simulink model "Intergration"  (R2018b)
settings: Solver=FixedStepDiscrete  StartTime=0.0  StopTime=inf  FixedStep=0.005  RelTol=1e-3
PostLoadFcn:
  | if any(exist('dsrtsu_mdlpostloadfcn', 'file') ~= 0), dsrtsu_mdlpostloadfcn('Execute', bdroot); end
values from neighbouring files (symbols this model uses):
  P_x165_On = 1.0    [CAN_Tx.sldd]
  P_x242_On = 1.0    [CAN_Tx.sldd]
  P_x246_On = 1.0    [CAN_Tx.sldd]
libraries: rtican x112, simulink x59
(part 4 of 31)

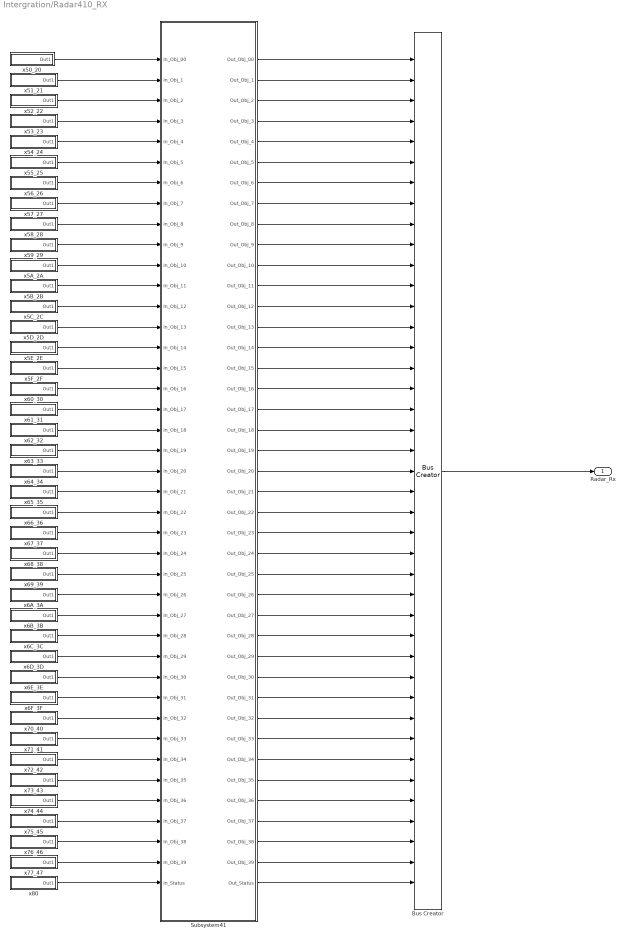
== system Intergration/Radar410_RX ==
  Bus Creator : BusCreator  Inputs=41  OutDataTypeStr=Bus: Radar410_Info_ST  NonVirtualBus=on
      settings: InheritFromInputs=off
  Subsystem41 : Subsystem
  x50_20 : Subsystem
  x51_21 : Subsystem
  x52_22 : Subsystem
  x53_23 : Subsystem
  x54_24 : Subsystem
  x55_25 : Subsystem
  x56_26 : Subsystem
  x57_27 : Subsystem
  x58_28 : Subsystem
  x59_29 : Subsystem
  x5A_2A : Subsystem
  x5B_2B : Subsystem
  x5C_2C : Subsystem
  x5D_2D : Subsystem
  x5E_2E : Subsystem
  x5F_2F : Subsystem
  x60_30 : Subsystem
  x61_31 : Subsystem
  x62_32 : Subsystem
  x63_33 : Subsystem
  x64_34 : Subsystem
  x65_35 : Subsystem
  x66_36 : Subsystem
  x67_37 : Subsystem
  x68_38 : Subsystem
  x69_39 : Subsystem
  x6A_3A : Subsystem
  x6B_3B : Subsystem
  x6C_3C : Subsystem
  x6D_3D : Subsystem
  x6E_3E : Subsystem
  x6F_3F : Subsystem
  x70_40 : Subsystem
  x71_41 : Subsystem
  x72_42 : Subsystem
  x73_43 : Subsystem
  x74_44 : Subsystem
  x75_45 : Subsystem
  x76_46 : Subsystem
  x77_47 : Subsystem
  x80 : Subsystem
  Radar_Rx : Outport  OutDataTypeStr=Bus: Radar410_Info_ST
  wires:
  Subsystem41/3(Out_Obj_2) -> Bus Creator/3
  x53_23/1(Out1) -> Subsystem41/4(In_Obj_3)
  x73_43/1(Out1) -> Subsystem41/36(In_Obj_35)
  x61_31/1(Out1) -> Subsystem41/18(In_Obj_17)
  x71_41/1(Out1) -> Subsystem41/34(In_Obj_33)
  x68_38/1(Out1) -> Subsystem41/25(In_Obj_24)
  Subsystem41/6(Out_Obj_5) -> Bus Creator/6
  Subsystem41/15(Out_Obj_14) -> Bus Creator/15
  Subsystem41/16(Out_Obj_15) -> Bus Creator/16
  Subsystem41/20(Out_Obj_19) -> Bus Creator/20
  x52_22/1(Out1) -> Subsystem41/3(In_Obj_2)
  Subsystem41/28(Out_Obj_27) -> Bus Creator/28
  Bus Creator/1 -> Radar_Rx/1
  Subsystem41/12(Out_Obj_11) -> Bus Creator/12
  x58_28/1(Out1) -> Subsystem41/9(In_Obj_8)
  Subsystem41/13(Out_Obj_12) -> Bus Creator/13
  Subsystem41/2(Out_Obj_1) -> Bus Creator/2
  x76_46/1(Out1) -> Subsystem41/39(In_Obj_38)
  Subsystem41/5(Out_Obj_4) -> Bus Creator/5
  x57_27/1(Out1) -> Subsystem41/8(In_Obj_7)
  x55_25/1(Out1) -> Subsystem41/6(In_Obj_5)
  x54_24/1(Out1) -> Subsystem41/5(In_Obj_4)
  x60_30/1(Out1) -> Subsystem41/17(In_Obj_16)
  x5A_2A/1(Out1) -> Subsystem41/11(In_Obj_10)
  Subsystem41/32(Out_Obj_31) -> Bus Creator/32
  x67_37/1(Out1) -> Subsystem41/24(In_Obj_23)
  x69_39/1(Out1) -> Subsystem41/26(In_Obj_25)
  x6C_3C/1(Out1) -> Subsystem41/29(In_Obj_28)
  x56_26/1(Out1) -> Subsystem41/7(In_Obj_6)
  x66_36/1(Out1) -> Subsystem41/23(In_Obj_22)
  x5F_2F/1(Out1) -> Subsystem41/16(In_Obj_15)
  x80/1(Out1) -> Subsystem41/41(In_Status)
  Subsystem41/41(Out_Status) -> Bus Creator/41
  x5E_2E/1(Out1) -> Subsystem41/15(In_Obj_14)
  x64_34/1(Out1) -> Subsystem41/21(In_Obj_20)
  x6F_3F/1(Out1) -> Subsystem41/32(In_Obj_31)
  x63_33/1(Out1) -> Subsystem41/20(In_Obj_19)
  Subsystem41/14(Out_Obj_13) -> Bus Creator/14
  x51_21/1(Out1) -> Subsystem41/2(In_Obj_1)
  Subsystem41/39(Out_Obj_38) -> Bus Creator/39
  x62_32/1(Out1) -> Subsystem41/19(In_Obj_18)
  x5B_2B/1(Out1) -> Subsystem41/12(In_Obj_11)
  Subsystem41/8(Out_Obj_7) -> Bus Creator/8
  Subsystem41/18(Out_Obj_17) -> Bus Creator/18
  Subsystem41/10(Out_Obj_9) -> Bus Creator/10
  x5C_2C/1(Out1) -> Subsystem41/13(In_Obj_12)
  Subsystem41/21(Out_Obj_20) -> Bus Creator/21
  x70_40/1(Out1) -> Subsystem41/33(In_Obj_32)
  x75_45/1(Out1) -> Subsystem41/38(In_Obj_37)
  x72_42/1(Out1) -> Subsystem41/35(In_Obj_34)
  Subsystem41/27(Out_Obj_26) -> Bus Creator/27
  Subsystem41/1(Out_Obj_00) -> Bus Creator/1
  x65_35/1(Out1) -> Subsystem41/22(In_Obj_21)
  Subsystem41/7(Out_Obj_6) -> Bus Creator/7
  Subsystem41/19(Out_Obj_18) -> Bus Creator/19
  Subsystem41/11(Out_Obj_10) -> Bus Creator/11
  x50_20/1(Out1) -> Subsystem41/1(In_Obj_00)
  x77_47/1(Out1) -> Subsystem41/40(In_Obj_39)
  x6B_3B/1(Out1) -> Subsystem41/28(In_Obj_27)
  Subsystem41/33(Out_Obj_32) -> Bus Creator/33
  Subsystem41/31(Out_Obj_30) -> Bus Creator/31
  Subsystem41/40(Out_Obj_39) -> Bus Creator/40
  x6A_3A/1(Out1) -> Subsystem41/27(In_Obj_26)
  Subsystem41/26(Out_Obj_25) -> Bus Creator/26
  Subsystem41/24(Out_Obj_23) -> Bus Creator/24
  x6D_3D/1(Out1) -> Subsystem41/30(In_Obj_29)
  Subsystem41/36(Out_Obj_35) -> Bus Creator/36
  Subsystem41/22(Out_Obj_21) -> Bus Creator/22
  Subsystem41/34(Out_Obj_33) -> Bus Creator/34
  Subsystem41/23(Out_Obj_22) -> Bus Creator/23
  Subsystem41/29(Out_Obj_28) -> Bus Creator/29
  Subsystem41/25(Out_Obj_24) -> Bus Creator/25
  Subsystem41/17(Out_Obj_16) -> Bus Creator/17
  Subsystem41/37(Out_Obj_36) -> Bus Creator/37
  x74_44/1(Out1) -> Subsystem41/37(In_Obj_36)
  x59_29/1(Out1) -> Subsystem41/10(In_Obj_9)
  x5D_2D/1(Out1) -> Subsystem41/14(In_Obj_13)
  Subsystem41/30(Out_Obj_29) -> Bus Creator/30
  Subsystem41/9(Out_Obj_8) -> Bus Creator/9
  Subsystem41/38(Out_Obj_37) -> Bus Creator/38
  Subsystem41/4(Out_Obj_3) -> Bus Creator/4
  x6E_3E/1(Out1) -> Subsystem41/31(In_Obj_30)
  Subsystem41/35(Out_Obj_34) -> Bus Creator/35

== system Intergration/TX ==
  VLC_LgtCmd_st : Inport  OutDataTypeStr=Bus: VLC_LGTCMD_ST  BusOutputAsStruct=on
  ACC_LgtCtrl_st : Inport  Port=2  OutDataTypeStr=Bus: ACC_LGTCTRL_ST  BusOutputAsStruct=on
  ATS_Po_st : Inport  Port=3  OutDataTypeStr=Bus: ATS_PO_ST
  COM_VehBus_st : Inport  Port=4
  do_20ms : TriggerPort  TriggerType=function-call  VariantControl=Variant
  Adapter_Tx : Subsystem
  Bus Selector : BusSelector  OutputSignals=x251.VehSdslSts,x24C.WhlGndVelLDrvn_Radar,x24C.WhlGndVelRDrvn_Radar,x24C.LDrvnWhlRotlDircn,x24C.RDrvnWhlRotlDircn,x24E.WhlGndVelLNonDrvn_Radar,x24E.WhlGndVelRNonDrvn_Radar,x24E.LNonDrvnWhlRotlDircn_Radar,x24E.RNonDrvnWhlRotlDircn_Radar,x23C.VehSpdAvg,x185.VSELongtAcc,x1E9.VehDynYawRate,x185.VSELatAcc
  Constant : Constant  Value=9.8
  Constant1 : Constant  Value=9.8
  Divide : Product  Inputs=*/
  Divide1 : Product  Inputs=*/
  ESC_DA_MESSAGE_0x127 : Subsystem
  ESC_FrontWheelSpeedKPH_0x123 : Subsystem
  ESC_RearWheelSpeedKPH_0x124 : Subsystem
  ESC_Status_0x126 : Subsystem
  RADAR_HSC2_FVCM_FrP00_0x165 : Subsystem
  RADAR_HSC2_FrP00_0x242 : Subsystem
  RADAR_HSC2_FrP01_0x244 : Subsystem
  RADAR_HSC2_FrP02_0x246 : Subsystem
  RollingCounter : Subsystem
  YRS1_0x131 : Subsystem
  YRS2_0x132 : Subsystem
  wires:
  VLC_LgtCmd_st/1 -> Adapter_Tx/1(VLC_LgtCmd_st)  "VLC_LgtCmd_st"
  RollingCounter/1(RC) -> RADAR_HSC2_FVCM_FrP00_0x165/1(RC), RADAR_HSC2_FrP01_0x244/1(RC), RADAR_HSC2_FrP00_0x242/1(RC)
  ATS_Po_st/1 -> Adapter_Tx/3(ATS_Po_st)
  ACC_LgtCtrl_st/1 -> Adapter_Tx/2(ACC_LgtCtrl_st)
  Adapter_Tx/3(x246) -> RADAR_HSC2_FrP02_0x246/1(COM_x246_st)
  Adapter_Tx/2(x165) -> RADAR_HSC2_FVCM_FrP00_0x165/2(COM_x165_st)  "COM_x165_st"
  Adapter_Tx/1(x242) -> RADAR_HSC2_FrP00_0x242/2(COM_x242_st)  "COM_x242_st"
  Bus Selector/8 -> ESC_RearWheelSpeedKPH_0x124/3(<LNonDrvnWhlRotlDircn_Radar>)  "<LNonDrvnWhlRotlDircn_Radar>"
  Constant/1 -> Divide/2
  Bus Selector/3 -> ESC_FrontWheelSpeedKPH_0x123/2(<WhlGndVelRDrvn_Radar>)  "<WhlGndVelRDrvn_Radar>"
  Constant1/1 -> Divide1/2
  Bus Selector/12 -> YRS1_0x131/1(<VehDynYawRate>)  "<VehDynYawRate>"
  COM_VehBus_st/1 -> Bus Selector/1
  Bus Selector/11 -> Divide/1  "<VSELongtAcc>"
  Divide1/1 -> YRS1_0x131/2(In2)
  Bus Selector/10 -> ESC_Status_0x126/1(<VehSpdAvg>)  "<VehSpdAvg>"
  Divide/1 -> YRS2_0x132/1(In1)
  Bus Selector/9 -> ESC_RearWheelSpeedKPH_0x124/4(<RNonDrvnWhlRotlDircn_Radar>)  "<RNonDrvnWhlRotlDircn_Radar>"
  Bus Selector/4 -> ESC_FrontWheelSpeedKPH_0x123/3(<LDrvnWhlRotlDircn>)  "<LDrvnWhlRotlDircn>"
  Bus Selector/13 -> Divide1/1  "<VSELatAcc>"
  Bus Selector/6 -> ESC_RearWheelSpeedKPH_0x124/1(<WhlGndVelLNonDrvn_Radar>)  "<WhlGndVelLNonDrvn_Radar>"
  Bus Selector/5 -> ESC_FrontWheelSpeedKPH_0x123/4(<RDrvnWhlRotlDircn>)  "<RDrvnWhlRotlDircn>"
  Bus Selector/7 -> ESC_RearWheelSpeedKPH_0x124/2(<WhlGndVelRNonDrvn_Radar>)  "<WhlGndVelRNonDrvn_Radar>"
  Bus Selector/2 -> ESC_FrontWheelSpeedKPH_0x123/1(<WhlGndVelLDrvn_Radar>)  "<WhlGndVelLDrvn_Radar>"
  Bus Selector/1 -> ESC_DA_MESSAGE_0x127/1(VehSdslStsHSC2)  "<VehSdslSts>"

== system Intergration/Tx_410_10ms ==
  COM_VehBus_st : Inport  OutDataTypeStr=Bus: COM_VEHBUS_ST  BusOutputAsStruct=on
  do_10ms : TriggerPort  TriggerType=function-call  VariantControl=Variant
  Abs : Abs
  Bus Selector1 : BusSelector  OutputSignals=x1E5.StrgWhlAngGrd,x1E5.StrgWhlAng
  Cast To Double{1..4} (4 alike) : DataTypeConversion  OutDataTypeStr=double
  Constant : Constant  Value=0  OutDataTypeStr=uint8
  Constant1 : Constant  Value=0  OutDataTypeStr=double
  Constant6 : Constant  Value=7  OutDataTypeStr=uint8
  RollingCounter1 : Subsystem
  S-Function Builder1 : S-Function  InitFcn=try, set_param(gcb,'FunctionName','CheckSum_Tx_Radar410'), end  FunctionName=CheckSum_Tx_Radar410  SFunctionModules=CheckSum_Tx_Radar410_wrapper  SFunctionDeploymentMode=off  EnableBusSupport=off  mask(S-Function Builder){}
      mask help: Simulink:masks:SFunctionBuilder_MD
      mask init:
      | val = [[.9  0.75 0.75 1 1 .9 .9 1]',[1 1 0.75 0.75 .9 .9 1 .9]'];try , sys = get_param(gcb,'SfunBuilderFcnName');if isempty(sys), sys = get_param(gcb,'FunctionName'); end,catch, sys = get_param(gcb,'FunctionName'); end
      settings: CopyFcn=set_param(gcbh,'LinkStatus','none')  PreSaveFcn=try, set_param(gcb,'FunctionName','CheckSum_Tx_Radar410'), end  OpenFcn=sfunctionwizard(gcbh)
      mask Display: plot(val(:,1),val(:,2)),disp(sys), port_label('input',1,'data'), port_label('input',2,'length'), port_label('output',1,'u8_crc8')
  SAS_Status : rtican/RTICAN Transmit (TX)   Reserved1=[]  Reserved2=[]  Reserved3=[]  Reserved4=[]  SfcnMessage=[]  Msg_Struct=[]  BoardTypeNo=[]  BoardNo=[]  ChannelNo=[]  Parameters=[]  DialogFcn=[]  UnitName=[]  Revision=[]  UnitValues=[]  DSProperties=struct('RTI',struct('Version',uint32(5),'BlockType',struct('isSLSource',uint8(1),'isSLSink',uint8(1),'isHWSource',uint8(0),'isHWSink',uint8(0),'isSetup',uint8(0),'isInline',uint8(1),'isNonInline',uint8(0),'isInterrupt',uint8(0),'isChannelwise',uint8(0)),'IOBoardType','RTICAN','UnitType','MESSAGE','Identifier','TX','DialogType','MSVC','BlockSet','RTICAN','SlaveProcessor','CAN'))  RTIBlockInterface=struct('InputPortsWidth',int32([1 1 1 1 1 1]),'InputPortsActive',[1 1 1 1 1 1],'InputPortsName',{{'SAS_Status_Checksum','SAS_Status_AliveCounter','SAS_CalibrationSts','SAS_FailureSts','SAS_SteerWheelRotSpd','SAS_SteerWheelAngle'}},'InputPortsDataType',{{'SS_DOUBLE','SS_DOUBLE','SS_DOUBLE','SS_DOUBLE','SS_DOUBLE','SS_DOUBLE'}},'OutputPortsWidth',int32([1 1 1 1]),'OutputPortsActive',[1 1 1 1],'OutputPortsName',{{['TX status'],['TX time'],['TX delta time'],['TX delay time']}},'DialogFcn','rtican_message_interface_gui','BlockDisplay',{{'','center'}},'IconTransparency','on','InitLevel',3,'BlockName',struct('Token',{{'SAS_Status'}}),'SampleTime',{{-1}},'TriggerPort',{{'none'}},'EnablePort',{{'none'}})  RTIBlockParameters=struct('BoardTypeNo',{{1,'OFF',[]}},'BoardNo',{{3,'ON',[1 16]}},'ChannelNo',{{2,'ON',[1 2]}},'Parameters',{{struct('DataFileSupport',struct('DataFileSelectedMaster',1,'DataFileSelectedLocal',1,'DataFileName','c:\users\administrator.zx-201607042142\documents\matlab\zone\dbc\ars410od_privatecan.dbc|c:\users\administrator.zx-201607042142\desktop\zone\2020_demo\410\asr410od_public_can.dbc|','DataFileDate',{{{''},{['30-十一月-2020 09:38:41']}}},'SelectedFile','..\..\..\..\..\desktop\zone\2020_demo\410\asr410od_public_can.dbc','InterfaceFcn','rtican_dbc_file_parser'),'Options',struct('StatusSelected',1,'TimeSelected',1,'DeltaTimeSelected',1,'DelayTimeSelected',1,'DelayTimeTXCommandSelected',0,'EncodeSetUnusedBitsToOne',0,'EnableMsgLoopback',0,'TriggerPort',struct('Selected',0,'TriggerType',0),'EnablePortSelected',0,'SignalOnPortnameSelected',1,'UserCoding',struct('Selected',0,'InterfaceFile','UserEncodingFile','FcnName','UserEncodeFcn','InportSelected',0,'InportWidth',1,'OutportSelected',0,'OutportWidth',1),'TerminationMsg',struct('Selected',0,'Byte0_7','0'),'InitialMsg',struct('Selected',0,'Byte0_7','0')),'Message',struct('MsgOnBlocknameSelected',1,'MsgName','SAS_Status','MsgIdFormat',0,'MsgId',225,'MsgLength',8,'NumSignals',6,'SampleTime',-1,'StartTime',struct('Selected',0,'Value',3),'AutoRepeatTime',struct('Selected',0,'Value',0.1),'Timeout',struct('Selected',0,'Value',0.1),'DelayTime',struct('Selected',0,'Value',0.1),'Signal',struct('SgnName',{'SAS_Status_Checksum','SAS_Status_AliveCounter','SAS_CalibrationSts','SAS_FailureSts','SAS_SteerWheelRotSpd','SAS_SteerWheelAngle'},'SgnStartBit',{16,28,38,39,40,48},'SgnLength',{8,4,1,1,8,16},'SgnType',{0,0,0,0,0,0},'ModeValue',{-1,-1,-1,-1,-1,-1},'DataType',{0,0,0,0,0,0},'ByteLayout',{2,2,2,2,2,2},'Factor',{1,1,1,1,4,0.1},'Offset',{0,0,0,0,0,-780},'SgnComment',{{'SAS_Status_Checksum'},{'SAS_Status_AliveCounter'},{'SAS_CalibrationSts'},{'SAS_FailureSts'},{'SAS_SteerWheelRotSpd'},{'SAS_SteerWheelAngle'}},'SgnUnit',{'','','','','',''},'Min',{0,0,0,0,0,-780},'Max',{255,15,1,1,1016,779.9},'SLDataType',{'SS_DOUBLE','SS_DOUBLE','SS_DOUBLE','SS_DOUBLE','SS_DOUBLE','SS_DOUBLE'}),'MsgIdNumFormat',1,'MsgComment',{{''}}),'Version',1.2,'general',struct('isFromLib',0)),'OFF',[]}},'GroupId',{{struct('Group',{{'RTICAN'}},'No',3,'Behavior',{{'NAMECHANGE'}},'BlockType',{{'SINK'}},'NameChangeFlag',0),'OFF',[]}},'SFcnRTICANMessage',{{struct('MsgType','TX','SFcnPortType','Scalar','MsgName','SAS_Status','MsgIdFormat','STD','MsgId',225,'MsgLength',8,'NumSignals',6,'SampleTime',-1,'StartTime',struct('Selected','no','Value',3),'AutoRepeatTime',struct('Selected','no','Value',0.1),'Timeout',struct('Selected','no','Value',0.1),'Signal',struct('SgnName',{'SAS_Status_Checksum','SAS_Status_AliveCounter','SAS_CalibrationSts','SAS_FailureSts','SAS_SteerWheelRotSpd','SAS_SteerWheelAngle'},'SgnStartBit',{16,28,38,39,40,48},'SgnLength',{8,4,1,1,8,16},'SgnType',{'standard','standard','standard','standard','standard','standard'},'ModeValue',{-1,-1,-1,-1,-1,-1},'DataType',{['unsigned int'],['unsigned int'],['unsigned int'],['unsigned int'],['unsigned int'],['unsigned int']},'ByteLayout',{['motorola back.'],['motorola back.'],['motorola back.'],['motorola back.'],['motorola back.'],['motorola back.']},'Factor',{1,1,1,1,4,0.1},'Offset',{0,0,0,0,0,-780},'SLDataType',{'SS_DOUBLE','SS_DOUBLE','SS_DOUBLE','SS_DOUBLE','SS_DOUBLE','SS_DOUBLE'}),'StatusSelected','yes','TimeSelected','yes','DeltaTimeSelected','yes','DelayTimeSelected','yes','DelayTimeTXCommandSelected','no','EncodeSetUnusedBitsToOne','no','EnableMsgLoopback','no','TriggerPort',struct('Selected','no','TriggerType',0),'EnablePortSelected','no','UserCoding',struct('Selected','no','InterfaceFile','UserEncodingFile','FcnName','UserEncodeFcn','InportSelected','no','InportWidth',1,'OutportSelected','no','OutportWidth',1),'TerminationMsg',struct('Selected','no','Byte0','0x00','Byte1','0x00','Byte2','0x00','Byte3','0x00','Byte4','0x00','Byte5','0x00','Byte6','0x00','Byte7','0x00'),'InitialMsg',struct('Selected','no','Byte0','0x00','Byte1','0x00','Byte2','0x00','Byte3','0x00','Byte4','0x00','Byte5','0x00','Byte6','0x00','Byte7','0x00'),'BoardType','DS1','BoardNo',3,'ControllerNo',2),'OFF',[]}},'TLCFileName',{{'rtican_tx_message','OFF',[]}})  RTISFcnParameters=struct('SFcnRTICANMessage','struct','TLCFileName','char')  RTIBlockParaDefault=struct('BoardTypeNo',4302,'BoardNo',1,'ChannelNo',1,'Parameters',struct('DataFileSupport',struct('DataFileSelectedMaster',0,'DataFileSelectedLocal',0,'DataFileName','','DataFileDate','','SelectedFile',['<no file selected>']),'Options',struct('StatusSelected',1,'TimeSelected',1,'DeltaTimeSelected',1,'DelayTimeSelected',1,'DelayTimeTXCommandSelected',0,'EncodeSetUnusedBitsToOne',0,'EnableMsgLoopback',0,'TriggerPort',struct('Selected',0,'TriggerType','rising'),'EnablePortSelected',0,'SignalOnPortnameSelected',1,'UserCoding',struct('Selected',0,'InterfaceFile','UserEncodingFile','FcnName','UserEncodeFcn','InportSelected',0,'InportWidth',1,'OutportSelected',0,'OutportWidth',1),'TerminationMsg',struct('Selected',0,'Byte0_7','0'),'InitialMsg',struct('Selected',0,'Byte0_7','0')),'Message',struct('MsgOnBlocknameSelected',0,'MsgName',['TX Message'],'MsgIdFormat',0,'MsgId',100,'MsgLength',8,'NumSignals',1,'SampleTime',-1,'StartTime',struct('Selected',0,'Value',0),'AutoRepeatTime',struct('Selected',0,'Value',0.1),'Timeout',struct('Selected',0,'Value',0.1),'DelayTime',struct('Selected',0,'Value',0.1),'Signal',struct('SgnName',['TX signal'],'SgnStartBit',0,'SgnLength',8,'SgnType',0,'ModeValue',-1,'DataType',0,'SLDataType','SS_DOUBLE','ByteLayout',0,'Factor',1,'Offset',0,'Min',0,'Max',255,'SgnComment',{{}},'SgnUnit',''),'MsgIdNumFormat',0,'MsgComment',{{''}}),'Version',1.2,'general',struct('isFromLib',1)),'GroupId',struct('Group',{{'RTICAN'}},'No',1,'Behavior',{{'NAMECHANGE'}},'BlockType',{{'SINK'}},'NameChangeFlag',0),'SFcnRTICANMessage',struct('MsgType','TX','MsgName',['TX Message'],'MsgIdFormat','STD','MsgId',100,'MsgLength',2,'NumSignals',1,'SampleTime',-1,'StartTime',struct('Selected','no','Value',0),'AutoRepeatTime',struct('Selected','no','Value',0.1),'Timeout',struct('Selected','no','Value',0.1),'DelayTime',struct('Selected','no','Value',0.1),'Signal',struct('SgnName',['TX signal'],'SgnStartBit',0,'SgnLength',8,'SgnType','standard','ModeValue',-1,'DataType',['unsigned int'],'ByteLayout',['little endian'],'SLDataType','SS_DOUBLE','Factor',1,'Offset',0),'StatusSelected','yes','TimeSelected','yes','DeltaTimeSelected','yes','DelayTimeSelected','yes','EnablePortSelected','no','EnableMsgLoopback','no','DelayTimeTXCommandSelected','no','EncodeSetUnusedBitsToOne','no','UserCoding',struct('Selected','no','InterfaceFile','UserDecodingFile','FcnName','UserDecodeFcn','InportSelected','no','InportWidth',1,'OutportSelected','no','OutportWidth',1),'TerminationMsg',struct('Selected','no','Byte0','0x00','Byte1','0x00','Byte2','0x00','Byte3','0x00','Byte4','0x00','Byte5','0x00','Byte6','0x00','Byte7','0x00'),'InitialMsg',struct('Selected','no','Byte0','0x00','Byte1','0x00','Byte2','0x00','Byte3','0x00','Byte4','0x00','Byte5','0x00','Byte6','0x00','Byte7','0x00'),'TriggerPort',struct('Selected','no','TriggerType','rising'),'BoardType','DS4302','BoardNo',1,'ControllerNo',1,'SFcnPortType','Scalar'),'TLCFileName','rtican_tx_message')
      settings: AttributesFormatString=Group Id: RTICAN3\n  SourceProductName=dSPACE RTI CAN Blockset
  Subsystem : Subsystem
  Subsystem1 : Subsystem
  Subsystem4 : Subsystem
  Vector Concatenate1 : Concatenate  NumInputs=7
  wires:
  Subsystem1/1(Byte0) -> Vector Concatenate1/1
  Cast To Double1/1 -> SAS_Status/5
  Cast To Double2/1 -> SAS_Status/6
  Subsystem4/1(Byte4) -> Vector Concatenate1/4, Cast To Double3/1
  Bus Selector1/1 -> Abs/1  "<StrgWhlAngGrd>"
  Constant1/1 -> SAS_Status/4, SAS_Status/3
  RollingCounter1/1(RC) -> Subsystem4/1(In1)
  Cast To Double3/1 -> SAS_Status/2
  Subsystem/1(Byte2) -> Vector Concatenate1/3
  Subsystem1/2(Out2) -> Cast To Double2/1
  Constant6/1 -> S-Function Builder1/2
  Cast To Double4/1 -> SAS_Status/1
  Subsystem1/3(Byte1) -> Vector Concatenate1/2
  Vector Concatenate1/1 -> S-Function Builder1/1
  Bus Selector1/2 -> Subsystem1/1(In1)  "<StrgWhlAng>"
  Abs/1 -> Cast To Double1/1, Subsystem/1(In1)
  COM_VehBus_st/1 -> Bus Selector1/1
  S-Function Builder1/1 -> Cast To Double4/1
  Constant/1 -> Vector Concatenate1/7, Vector Concatenate1/6, Vector Concatenate1/5

== system Intergration/RTI Data/RTI Data Store ==
  RTI Data Store : Subsystem  mask(RTI_DATA_STORE){}
      mask help:
      | RTI Data Store Block. This block is used by RTI to store internal model dependent data. Deleting this block will result in data loss.
      |
      | NEVER DELETE, COPY, OR MODIFY THIS BLOCK!
      mask Help:
      | RTI Data Store Block. This block is used by RTI to store internal model dependent data. Deleting this block will result in data loss.
      | 
      | NEVER DELETE, COPY, OR MODIFY THIS BLOCK!
      mask Display: text(0.5, 0.5, ' ', 'HorizontalAlignment', 'center');

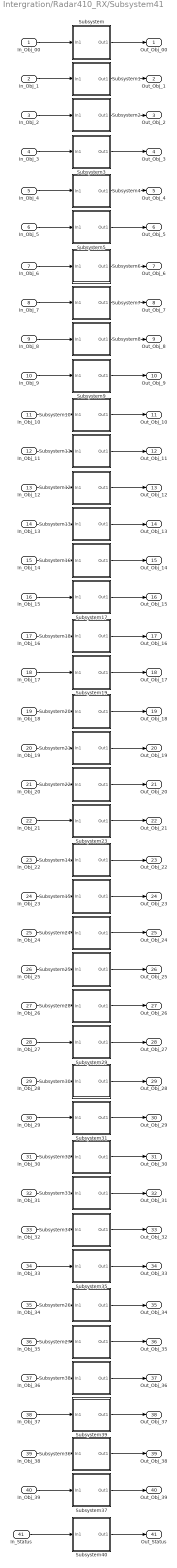
== system Intergration/Radar410_RX/Subsystem41 ==
  In_Obj_00 : Inport
  In_Obj_1 : Inport  Port=2
  In_Obj_2 : Inport  Port=3
  In_Obj_3 : Inport  Port=4
  In_Obj_4 : Inport  Port=5
  In_Obj_5 : Inport  Port=6
  In_Obj_6 : Inport  Port=7
  In_Obj_7 : Inport  Port=8
  In_Obj_8 : Inport  Port=9
  In_Obj_9 : Inport  Port=10
  In_Obj_10 : Inport  Port=11
  In_Obj_11 : Inport  Port=12
  In_Obj_12 : Inport  Port=13
  In_Obj_13 : Inport  Port=14
  In_Obj_14 : Inport  Port=15
  In_Obj_15 : Inport  Port=16
  In_Obj_16 : Inport  Port=17
  In_Obj_17 : Inport  Port=18
  In_Obj_18 : Inport  Port=19
  In_Obj_19 : Inport  Port=20
  In_Obj_20 : Inport  Port=21
  In_Obj_21 : Inport  Port=22
  In_Obj_22 : Inport  Port=23
  In_Obj_23 : Inport  Port=24
  In_Obj_24 : Inport  Port=25
  In_Obj_25 : Inport  Port=26
  In_Obj_26 : Inport  Port=27
  In_Obj_27 : Inport  Port=28
  In_Obj_28 : Inport  Port=29
  In_Obj_29 : Inport  Port=30
  In_Obj_30 : Inport  Port=31
  In_Obj_31 : Inport  Port=32
  In_Obj_32 : Inport  Port=33
  In_Obj_33 : Inport  Port=34
  In_Obj_34 : Inport  Port=35
  In_Obj_35 : Inport  Port=36
  In_Obj_36 : Inport  Port=37
  In_Obj_37 : Inport  Port=38
  In_Obj_38 : Inport  Port=39
  In_Obj_39 : Inport  Port=40
  In_Status : Inport  Port=41
  Subsystem : Subsystem
  Subsystem1 : Subsystem
  Subsystem10 : Subsystem
  Subsystem11 : Subsystem
  Subsystem12 : Subsystem
  Subsystem13 : Subsystem
  Subsystem14 : Subsystem
  Subsystem15 : Subsystem
  Subsystem16 : Subsystem
  Subsystem17 : Subsystem
  Subsystem18 : Subsystem
  Subsystem19 : Subsystem
  Subsystem2 : Subsystem
  Subsystem20 : Subsystem
  Subsystem21 : Subsystem
  Subsystem22 : Subsystem
  Subsystem23 : Subsystem
  Subsystem24 : Subsystem
  Subsystem25 : Subsystem
  Subsystem26 : Subsystem
  Subsystem27 : Subsystem
  Subsystem28 : Subsystem
  Subsystem29 : Subsystem
  Subsystem3 : Subsystem
  Subsystem30 : Subsystem
  Subsystem31 : Subsystem
  Subsystem32 : Subsystem
  Subsystem33 : Subsystem
  Subsystem34 : Subsystem
  Subsystem35 : Subsystem
  Subsystem36 : Subsystem
  Subsystem37 : Subsystem
  Subsystem38 : Subsystem
  Subsystem39 : Subsystem
  Subsystem4 : Subsystem
  Subsystem40 : Subsystem
  Subsystem5 : Subsystem
  Subsystem6 : Subsystem
  Subsystem7 : Subsystem
  Subsystem8 : Subsystem
  Subsystem9 : Subsystem
  Out_Obj_00 : Outport  OutDataTypeStr=Bus: Obj_Data
  Out_Obj_1 : Outport  Port=2  OutDataTypeStr=Bus: Obj_Data
  Out_Obj_2 : Outport  Port=3  OutDataTypeStr=Bus: Obj_Data
  Out_Obj_3 : Outport  Port=4  OutDataTypeStr=Bus: Obj_Data
  Out_Obj_4 : Outport  Port=5  OutDataTypeStr=Bus: Obj_Data
  Out_Obj_5 : Outport  Port=6  OutDataTypeStr=Bus: Obj_Data
  Out_Obj_6 : Outport  Port=7  OutDataTypeStr=Bus: Obj_Data
  Out_Obj_7 : Outport  Port=8  OutDataTypeStr=Bus: Obj_Data
  Out_Obj_8 : Outport  Port=9  OutDataTypeStr=Bus: Obj_Data
  Out_Obj_9 : Outport  Port=10  OutDataTypeStr=Bus: Obj_Data
  Out_Obj_10 : Outport  Port=11  OutDataTypeStr=Bus: Obj_Data
  Out_Obj_11 : Outport  Port=12  OutDataTypeStr=Bus: Obj_Data
  Out_Obj_12 : Outport  Port=13  OutDataTypeStr=Bus: Obj_Data
  Out_Obj_13 : Outport  Port=14  OutDataTypeStr=Bus: Obj_Data
  Out_Obj_14 : Outport  Port=15  OutDataTypeStr=Bus: Obj_Data
  Out_Obj_15 : Outport  Port=16  OutDataTypeStr=Bus: Obj_Data
  Out_Obj_16 : Outport  Port=17  OutDataTypeStr=Bus: Obj_Data
  Out_Obj_17 : Outport  Port=18  OutDataTypeStr=Bus: Obj_Data
  Out_Obj_18 : Outport  Port=19  OutDataTypeStr=Bus: Obj_Data
  Out_Obj_19 : Outport  Port=20  OutDataTypeStr=Bus: Obj_Data
  Out_Obj_20 : Outport  Port=21  OutDataTypeStr=Bus: Obj_Data
  Out_Obj_21 : Outport  Port=22  OutDataTypeStr=Bus: Obj_Data
  Out_Obj_22 : Outport  Port=23  OutDataTypeStr=Bus: Obj_Data
  Out_Obj_23 : Outport  Port=24  OutDataTypeStr=Bus: Obj_Data
  Out_Obj_24 : Outport  Port=25  OutDataTypeStr=Bus: Obj_Data
  Out_Obj_25 : Outport  Port=26  OutDataTypeStr=Bus: Obj_Data
  Out_Obj_26 : Outport  Port=27  OutDataTypeStr=Bus: Obj_Data
  Out_Obj_27 : Outport  Port=28  OutDataTypeStr=Bus: Obj_Data
  Out_Obj_28 : Outport  Port=29  OutDataTypeStr=Bus: Obj_Data
  Out_Obj_29 : Outport  Port=30  OutDataTypeStr=Bus: Obj_Data
  Out_Obj_30 : Outport  Port=31  OutDataTypeStr=Bus: Obj_Data
  Out_Obj_31 : Outport  Port=32  OutDataTypeStr=Bus: Obj_Data
  Out_Obj_32 : Outport  Port=33  OutDataTypeStr=Bus: Obj_Data
  Out_Obj_33 : Outport  Port=34  OutDataTypeStr=Bus: Obj_Data
  Out_Obj_34 : Outport  Port=35  OutDataTypeStr=Bus: Obj_Data
  Out_Obj_35 : Outport  Port=36  OutDataTypeStr=Bus: Obj_Data
  Out_Obj_36 : Outport  Port=37  OutDataTypeStr=Bus: Obj_Data
  Out_Obj_37 : Outport  Port=38  OutDataTypeStr=Bus: Obj_Data
  Out_Obj_38 : Outport  Port=39  OutDataTypeStr=Bus: Obj_Data
  Out_Obj_39 : Outport  Port=40  OutDataTypeStr=Bus: Obj_Data
  Out_Status : Outport  Port=41  OutDataTypeStr=Bus: Radar_Status
  wires:
  In_Status/1 -> Subsystem40/1(In1)
  In_Obj_00/1 -> Subsystem/1(In1)
  Subsystem40/1(Out1) -> Out_Status/1
  Subsystem/1(Out1) -> Out_Obj_00/1
  Subsystem1/1(Out1) -> Out_Obj_1/1
  In_Obj_1/1 -> Subsystem1/1(In1)
  In_Obj_3/1 -> Subsystem3/1(In1)
  Subsystem3/1(Out1) -> Out_Obj_3/1
  Subsystem2/1(Out1) -> Out_Obj_2/1
  In_Obj_2/1 -> Subsystem2/1(In1)
  In_Obj_4/1 -> Subsystem4/1(In1)
  Subsystem4/1(Out1) -> Out_Obj_4/1
  Subsystem5/1(Out1) -> Out_Obj_5/1
  In_Obj_5/1 -> Subsystem5/1(In1)
  In_Obj_11/1 -> Subsystem11/1(In1)
  Subsystem11/1(Out1) -> Out_Obj_11/1
  Subsystem10/1(Out1) -> Out_Obj_10/1
  In_Obj_10/1 -> Subsystem10/1(In1)
  In_Obj_8/1 -> Subsystem8/1(In1)
  Subsystem8/1(Out1) -> Out_Obj_8/1
  Subsystem9/1(Out1) -> Out_Obj_9/1
  In_Obj_9/1 -> Subsystem9/1(In1)
  In_Obj_7/1 -> Subsystem7/1(In1)
  Subsystem7/1(Out1) -> Out_Obj_7/1
  Subsystem6/1(Out1) -> Out_Obj_6/1
  In_Obj_6/1 -> Subsystem6/1(In1)
  In_Obj_18/1 -> Subsystem20/1(In1)
  Subsystem20/1(Out1) -> Out_Obj_18/1
  Subsystem21/1(Out1) -> Out_Obj_19/1
  In_Obj_19/1 -> Subsystem21/1(In1)
  In_Obj_21/1 -> Subsystem23/1(In1)
  Subsystem23/1(Out1) -> Out_Obj_21/1
  Subsystem22/1(Out1) -> Out_Obj_20/1
  In_Obj_20/1 -> Subsystem22/1(In1)
  In_Obj_22/1 -> Subsystem14/1(In1)
  Subsystem14/1(Out1) -> Out_Obj_22/1
  Subsystem15/1(Out1) -> Out_Obj_23/1
  In_Obj_23/1 -> Subsystem15/1(In1)
  In_Obj_17/1 -> Subsystem19/1(In1)
  Subsystem19/1(Out1) -> Out_Obj_17/1
  Subsystem18/1(Out1) -> Out_Obj_16/1
  In_Obj_16/1 -> Subsystem18/1(In1)
  In_Obj_14/1 -> Subsystem16/1(In1)
  Subsystem16/1(Out1) -> Out_Obj_14/1
  Subsystem17/1(Out1) -> Out_Obj_15/1
  In_Obj_15/1 -> Subsystem17/1(In1)
  In_Obj_13/1 -> Subsystem13/1(In1)
  Subsystem13/1(Out1) -> Out_Obj_13/1
  Subsystem12/1(Out1) -> Out_Obj_12/1
  In_Obj_12/1 -> Subsystem12/1(In1)
  In_Obj_24/1 -> Subsystem24/1(In1)
  Subsystem24/1(Out1) -> Out_Obj_24/1
  Subsystem25/1(Out1) -> Out_Obj_25/1
  In_Obj_25/1 -> Subsystem25/1(In1)
  In_Obj_27/1 -> Subsystem29/1(In1)
  Subsystem29/1(Out1) -> Out_Obj_27/1
  Subsystem28/1(Out1) -> Out_Obj_26/1
  In_Obj_26/1 -> Subsystem28/1(In1)
  In_Obj_28/1 -> Subsystem30/1(In1)
  Subsystem30/1(Out1) -> Out_Obj_28/1
  Subsystem31/1(Out1) -> Out_Obj_29/1
  In_Obj_29/1 -> Subsystem31/1(In1)
  In_Obj_35/1 -> Subsystem27/1(In1)
  Subsystem27/1(Out1) -> Out_Obj_35/1
  Subsystem26/1(Out1) -> Out_Obj_34/1
  In_Obj_34/1 -> Subsystem26/1(In1)
  In_Obj_32/1 -> Subsystem34/1(In1)
  Subsystem34/1(Out1) -> Out_Obj_32/1
  Subsystem35/1(Out1) -> Out_Obj_33/1
  In_Obj_33/1 -> Subsystem35/1(In1)
  In_Obj_31/1 -> Subsystem33/1(In1)
  Subsystem33/1(Out1) -> Out_Obj_31/1
  Subsystem32/1(Out1) -> Out_Obj_30/1
  In_Obj_30/1 -> Subsystem32/1(In1)
  In_Obj_37/1 -> Subsystem39/1(In1)
  Subsystem39/1(Out1) -> Out_Obj_37/1
  Subsystem38/1(Out1) -> Out_Obj_36/1
  In_Obj_36/1 -> Subsystem38/1(In1)
  In_Obj_38/1 -> Subsystem36/1(In1)
  Subsystem36/1(Out1) -> Out_Obj_38/1
  Subsystem37/1(Out1) -> Out_Obj_39/1
  In_Obj_39/1 -> Subsystem37/1(In1)

== system Intergration/Radar410_RX/x50_20 ==
  Bus Creator1 : BusCreator  Inputs=20
  FRS_Obj_00_Part1of2 : rtican/RTICAN Receive (RX)   Reserved1=[]  Reserved2=[]  Reserved3=[]  Reserved4=[]  SfcnMessage=[]  Msg_Struct=[]  BoardTypeNo=[]  BoardNo=[]  ChannelNo=[]  Parameters=[]  DialogFcn=[]  UnitName=[]  Revision=[]  UnitValues=[]  DSProperties=struct('RTI',struct('Version',uint32(5),'BlockType',struct('isSLSource',uint8(1),'isSLSink',uint8(1),'isHWSource',uint8(0),'isHWSink',uint8(0),'isSetup',uint8(0),'isInline',uint8(1),'isNonInline',uint8(0),'isInterrupt',uint8(0),'isChannelwise',uint8(0)),'IOBoardType','RTICAN','UnitType','MESSAGE','Identifier','RX','DialogType','MSVC','BlockSet','RTICAN','SlaveProcessor','CAN'))  RTIBlockInterface=struct('OutputPortsWidth',int32([1 1 1 1 1 1 1 1 1 1 1 1 1 1 1]),'OutputPortsActive',ones(1,15),'OutputPortsName',{{'FRS_P1_00_Msg_CheckSum','FRS_P1_00_Msg_AliveCounter','FRS_P1_00_Obj_ExstProb','FRS_P1_00_Obj_XVelRel_Stdev','FRS_P1_00_Obj_XAccRel','FRS_P1_00_Obj_ObstacleProb','FRS_P1_00_Obj_MotionPattern','FRS_P1_00_Obj_YPos_Stdev','FRS_P1_00_Obj_ValidFlag','FRS_P1_00_Obj_XPos_Stdev','FRS_P1_00_Obj_UpdateFlag','FRS_P1_00_Obj_ID',['RX status'],['RX time'],['RX delta time']}},'OutputPortsDataType',{{'SS_DOUBLE','SS_DOUBLE','SS_DOUBLE','SS_DOUBLE','SS_DOUBLE','SS_DOUBLE','SS_DOUBLE','SS_DOUBLE','SS_DOUBLE','SS_DOUBLE','SS_DOUBLE','SS_DOUBLE','SS_DOUBLE','SS_DOUBLE','SS_DOUBLE'}},'OutputPortsLabel',{{'FRS_P1_00_Msg_CheckSum','FRS_P1_00_Msg_AliveCounter','FRS_P1_00_Obj_ExstProb','FRS_P1_00_Obj_XVelRel_Stdev','FRS_P1_00_Obj_XAccRel','FRS_P1_00_Obj_ObstacleProb','FRS_P1_00_Obj_MotionPattern','FRS_P1_00_Obj_YPos_Stdev','FRS_P1_00_Obj_ValidFlag','FRS_P1_00_Obj_XPos_Stdev','FRS_P1_00_Obj_UpdateFlag','FRS_P1_00_Obj_ID','','',''}},'OutputPortsLabelMode','ON','InputPortsWidth',int32(0),'InputPortsActive',0,'DialogFcn','rtican_message_interface_gui','BlockDisplay',{{'','center'}},'IconTransparency','on','ParameterTunableNames',{{}},'InitLevel',3,'BlockName',struct('Token',{{'FRS_Obj_00_Part1of2'}}),'SampleTime',{{-1}},'TriggerPort',{{'none'}},'EnablePort',{{'none'}})  RTIBlockParameters=struct('BoardTypeNo',{{1,'OFF',[]}},'BoardNo',{{2,'ON',[1 16]}},'ChannelNo',{{2,'ON',[1 2]}},'Parameters',{{struct('DataFileSupport',struct('DataFileSelectedMaster',1,'DataFileSelectedLocal',1,'DataFileName','d:\00_work\00_zop\00_zop_demo_sim\asr410od_privatecan\privatecan\ars410od_privatecan.dbc|','DataFileDate',{{{['04-12月-2019 16:27:24']}}},'SelectedFile','asr410od_privatecan\privatecan\ars410od_privatecan.dbc'),'Options',struct('StatusSelected',1,'TimeSelected',1,'DeltaTimeSelected',1,'BytePortSelected',0,'MessageLengthSelected',0,'TriggerPort',struct('Selected',0,'TriggerType',0),'UserCoding',struct('Selected',0,'InterfaceFile','UserDecodingFile','FcnName','UserDecodeFcn','InportSelected',0,'InportWidth',1,'OutportSelected',0,'OutportWidth',1),'EnablePortSelected',0,'SignalOnPortnameSelected',1,'UseRXService',0),'Message',struct('MsgOnBlocknameSelected',1,'MsgName','FRS_Obj_00_Part1of2','MsgIdFormat',0,'MsgId',80,'MsgLength',8,'NumSignals',12,'SampleTime',-1,'Signal',struct('SgnName',{'FRS_P1_00_Msg_CheckSum','FRS_P1_00_Msg_AliveCounter','FRS_P1_00_Obj_ExstProb','FRS_P1_00_Obj_XVelRel_Stdev','FRS_P1_00_Obj_XAccRel','FRS_P1_00_Obj_ObstacleProb','FRS_P1_00_Obj_MotionPattern','FRS_P1_00_Obj_YPos_Stdev','FRS_P1_00_Obj_ValidFlag','FRS_P1_00_Obj_XPos_Stdev','FRS_P1_00_Obj_UpdateFlag','FRS_P1_00_Obj_ID'},'SgnStartBit',{0,8,12,18,25,32,37,40,47,48,55,56},'SgnLength',{8,4,6,7,7,5,3,7,1,7,1,8},'SgnType',{0,0,0,0,0,0,0,0,0,0,0,0},'ModeValue',{-1,-1,-1,-1,-1,-1,-1,-1,-1,-1,-1,-1},'DataType',{0,0,0,0,0,0,0,0,0,0,0,0},'ByteLayout',{2,2,2,2,2,2,2,2,2,2,2,2},'Factor',{1,1,1.5873,0.05,0.15,3.2258,1,0.1,1,0.1,1,1},'Offset',{0,0,0,0,-9.6,0,0,0,0,0,0,0},'SgnComment',{{['Check sum shall be generated out of each message content. check sum generation logic is TBC.']},{['Alive counter shall be incremented every radar sensor measurement cycle.']},{['Estimated existence probability of the object.']},{['Estimated 3-sigma standard deviation value of the relative longitudinal velocity of the object.']},{['Relative longitudinal acceleration of the object']},{['Estimated probability of the object being an obstacle.']},{['Motion type of object.' char(10) '0x00: Unknown' char(10) '0x01: Stationary' char(10) '0x02: Stopped' char(10) '0x03: Moving' char(10) '0x04: Crossing' char(10) '0x05-07: reserved']},{['Estimated 3-sigma standard deviation value of lateral position of the object.']},{['Validity indication flag. when this value shows invalid, all the signals in the corresponding CAN messages except FRS_Msg_AliveCounter and FRS_Msg_CheckSum shall take default values.' char(10) '0x0: Object invalid' char(10) '0x1: Object valid']},{['Estimated 3-sigma standard deviation value of longitudinal position of the object.']},{['Flag to indicate newly created object in CAN bus.' char(10) 'Object history flag' char(10) '0x0: new object in the cycle;' char(10) '0x1: object existed in previous cycle']},{['ID is defined as a unique identification number over the lifetime of the object.' char(10) '0xFF: Invalid' char(10) '0x00 - 0xFE: Valid']}},'SgnUnit',{'n/a','n/a','%','m/s','m/s2','%','n/a','m','n/a','m','n/a','n/a'},'Min',{0,0,0,0,-9.6,0,0,0,0,0,0,0},'Max',{255,15,99.9999,6.35,9.45,99.9998,7,12.7,1,12.7,1,255},'SLDataType',{'SS_DOUBLE','SS_DOUBLE','SS_DOUBLE','SS_DOUBLE','SS_DOUBLE','SS_DOUBLE','SS_DOUBLE','SS_DOUBLE','SS_DOUBLE','SS_DOUBLE','SS_DOUBLE','SS_DOUBLE'}),'MsgIdNumFormat',1,'MsgComment',{{''}}),'Version',1.2,'general',struct('isFromLib',0)),'OFF',[]}},'GroupId',{{struct('Group',{{'RTICAN'}},'No',2,'Behavior',{{'NAMECHANGE'}},'BlockType',{{'SINK'}},'NameChangeFlag',0),'OFF',[]}},'SFcnRTICANMessage',{{struct('MsgType','RX','SFcnPortType','Scalar','MsgName','FRS_Obj_00_Part1of2','MsgIdFormat','STD','MsgId',80,'MsgLength',8,'NumSignals',12,'SampleTime',-1,'Signal',struct('SgnName',{'FRS_P1_00_Msg_CheckSum','FRS_P1_00_Msg_AliveCounter','FRS_P1_00_Obj_ExstProb','FRS_P1_00_Obj_XVelRel_Stdev','FRS_P1_00_Obj_XAccRel','FRS_P1_00_Obj_ObstacleProb','FRS_P1_00_Obj_MotionPattern','FRS_P1_00_Obj_YPos_Stdev','FRS_P1_00_Obj_ValidFlag','FRS_P1_00_Obj_XPos_Stdev','FRS_P1_00_Obj_UpdateFlag','FRS_P1_00_Obj_ID'},'SgnStartBit',{0,8,12,18,25,32,37,40,47,48,55,56},'SgnLength',{8,4,6,7,7,5,3,7,1,7,1,8},'SgnType',{'standard','standard','standard','standard','standard','standard','standard','standard','standard','standard','standard','standard'},'ModeValue',{-1,-1,-1,-1,-1,-1,-1,-1,-1,-1,-1,-1},'DataType',{['unsigned int'],['unsigned int'],['unsigned int'],['unsigned int'],['unsigned int'],['unsigned int'],['unsigned int'],['unsigned int'],['unsigned int'],['unsigned int'],['unsigned int'],['unsigned int']},'ByteLayout',{['motorola back.'],['motorola back.'],['motorola back.'],['motorola back.'],['motorola back.'],['motorola back.'],['motorola back.'],['motorola back.'],['motorola back.'],['motorola back.'],['motorola back.'],['motorola back.']},'Factor',{1,1,1.5873,0.05,0.15,3.2258,1,0.1,1,0.1,1,1},'Offset',{0,0,0,0,-9.6,0,0,0,0,0,0,0},'SLDataType',{'SS_DOUBLE','SS_DOUBLE','SS_DOUBLE','SS_DOUBLE','SS_DOUBLE','SS_DOUBLE','SS_DOUBLE','SS_DOUBLE','SS_DOUBLE','SS_DOUBLE','SS_DOUBLE','SS_DOUBLE'}),'StatusSelected','yes','TimeSelected','yes','DeltaTimeSelected','yes','BytePortSelected','no','MessageLengthSelected','no','TriggerPort',struct('Selected','no','TriggerType',0),'UserCoding',struct('Selected','no','InterfaceFile','UserDecodingFile','FcnName','UserDecodeFcn','InportSelected','no','InportWidth',1,'OutportSelected','no','OutportWidth',1),'EnablePortSelected','no','UseRXService','no','BoardType','DS1','BoardNo',2,'ControllerNo',1),'OFF',[]}},'TLCFileName',{{'rtican_rx_message','OFF',[]}})  RTISFcnParameters=struct('SFcnRTICANMessage','struct','TLCFileName','char')  RTIBlockParaDefault=struct('BoardTypeNo',4302,'BoardNo',1,'ChannelNo',1,'Parameters',struct('DataFileSupport',struct('DataFileSelectedMaster',0,'DataFileSelectedLocal',0,'DataFileName','','DataFileDate','','SelectedFile',['<no file selected>']),'Options',struct('StatusSelected',1,'TimeSelected',1,'DeltaTimeSelected',1,'BytePortSelected',0,'MessageLengthSelected',0,'TriggerPort',struct('Selected',0,'TriggerType','rising'),'UserCoding',struct('Selected',0,'InterfaceFile','UserDecodingFile','FcnName','UserDecodeFcn','InportSelected',0,'InportWidth',1,'OutportSelected',0,'OutportWidth',1),'EnablePortSelected',0,'SignalOnPortnameSelected',1,'UseRXService',0),'Message',struct('MsgOnBlocknameSelected',0,'MsgName',['RX Message'],'MsgIdFormat',0,'MsgId',100,'MsgLength',8,'NumSignals',1,'SampleTime',-1,'Signal',struct('SgnName',['RX signal'],'SgnStartBit',0,'SgnLength',8,'SgnType',0,'ModeValue',-1,'DataType',0,'SLDataType','SS_DOUBLE','ByteLayout',0,'Factor',1,'Offset',0,'Min',0,'Max',255,'SgnComment',{{}},'SgnUnit',''),'MsgIdNumFormat',0,'MsgComment',{{''}}),'Version',1.2,'general',struct('isFromLib',1)),'GroupId',struct('Group',{{'RTICAN'}},'No',1,'Behavior',{{'NAMECHANGE'}},'BlockType',{{'SINK'}},'NameChangeFlag',0),'SFcnRTICANMessage',struct('MsgType','RX','MsgName',['RX Message'],'MsgIdFormat','STD','MsgId',100,'MsgLength',8,'NumSignals',1,'SampleTime',-1,'Signal',struct('SgnName',['RX signal'],'SgnStartBit',0,'SgnLength',8,'SgnType','standard','ModeValue',-1,'DataType',['unsigned int'],'ByteLayout',['little endian'],'SLDataType','SS_DOUBLE','Factor',1,'Offset',0),'StatusSelected','yes','TimeSelected','yes','DeltaTimeSelected','yes','BytePortSelected','no','MessageLengthSelected','no','EnablePortSelected','no','UserCoding',struct('Selected','no','InterfaceFile','UserDecodingFile','FcnName','UserDecodeFcn','InportSelected','no','InportWidth',1,'OutportSelected','no','OutportWidth',1),'TriggerPort',struct('Selected','no','TriggerType','rising'),'UseRXService','no','BoardType','DS4302','BoardNo',1,'ControllerNo',1,'SFcnPortType','Scalar'),'TLCFileName','rtican_rx_message')
      settings: AttributesFormatString=Group Id: RTICAN2\n  SourceProductName=dSPACE RTI CAN Blockset
  FRS_Obj_00_Part2of2 : rtican/RTICAN Receive (RX)   Reserved1=[]  Reserved2=[]  Reserved3=[]  Reserved4=[]  SfcnMessage=[]  Msg_Struct=[]  BoardTypeNo=[]  BoardNo=[]  ChannelNo=[]  Parameters=[]  DialogFcn=[]  UnitName=[]  Revision=[]  UnitValues=[]  DSProperties=struct('RTI',struct('Version',uint32(5),'BlockType',struct('isSLSource',uint8(1),'isSLSink',uint8(1),'isHWSource',uint8(0),'isHWSink',uint8(0),'isSetup',uint8(0),'isInline',uint8(1),'isNonInline',uint8(0),'isInterrupt',uint8(0),'isChannelwise',uint8(0)),'IOBoardType','RTICAN','UnitType','MESSAGE','Identifier','RX','DialogType','MSVC','BlockSet','RTICAN','SlaveProcessor','CAN'))  RTIBlockInterface=struct('OutputPortsWidth',int32([1 1 1 1 1 1 1 1 1 1 1]),'OutputPortsActive',ones(1,11),'OutputPortsName',{{'FRS_P2_00_Msg_CheckSum','FRS_P2_00_Msg_AliveCounter','FRS_P2_00_Obj_MeasFlag','FRS_P2_00_Obj_YVelRel','FRS_P2_00_Obj_Type','FRS_P2_00_Obj_XPos','FRS_P2_00_Obj_YPos','FRS_P2_00_Obj_XVelRel',['RX status'],['RX time'],['RX delta time']}},'OutputPortsDataType',{{'SS_DOUBLE','SS_DOUBLE','SS_DOUBLE','SS_DOUBLE','SS_DOUBLE','SS_DOUBLE','SS_DOUBLE','SS_DOUBLE','SS_DOUBLE','SS_DOUBLE','SS_DOUBLE'}},'OutputPortsLabel',{{'FRS_P2_00_Msg_CheckSum','FRS_P2_00_Msg_AliveCounter','FRS_P2_00_Obj_MeasFlag','FRS_P2_00_Obj_YVelRel','FRS_P2_00_Obj_Type','FRS_P2_00_Obj_XPos','FRS_P2_00_Obj_YPos','FRS_P2_00_Obj_XVelRel','','',''}},'OutputPortsLabelMode','ON','InputPortsWidth',int32(0),'InputPortsActive',0,'DialogFcn','rtican_message_interface_gui','BlockDisplay',{{'','center'}},'IconTransparency','on','ParameterTunableNames',{{}},'InitLevel',3,'BlockName',struct('Token',{{'FRS_Obj_00_Part2of2'}}),'SampleTime',{{-1}},'TriggerPort',{{'none'}},'EnablePort',{{'none'}})  RTIBlockParameters=struct('BoardTypeNo',{{1,'OFF',[]}},'BoardNo',{{2,'ON',[1 16]}},'ChannelNo',{{2,'ON',[1 2]}},'Parameters',{{struct('DataFileSupport',struct('DataFileSelectedMaster',1,'DataFileSelectedLocal',1,'DataFileName','d:\00_work\00_zop\00_zop_demo_sim\asr410od_privatecan\privatecan\ars410od_privatecan.dbc|','DataFileDate',{{{['04-12月-2019 16:27:24']}}},'SelectedFile','asr410od_privatecan\privatecan\ars410od_privatecan.dbc'),'Options',struct('StatusSelected',1,'TimeSelected',1,'DeltaTimeSelected',1,'BytePortSelected',0,'MessageLengthSelected',0,'TriggerPort',struct('Selected',0,'TriggerType',0),'UserCoding',struct('Selected',0,'InterfaceFile','UserDecodingFile','FcnName','UserDecodeFcn','InportSelected',0,'InportWidth',1,'OutportSelected',0,'OutportWidth',1),'EnablePortSelected',0,'SignalOnPortnameSelected',1,'UseRXService',0),'Message',struct('MsgOnBlocknameSelected',1,'MsgName','FRS_Obj_00_Part2of2','MsgIdFormat',0,'MsgId',32,'MsgLength',8,'NumSignals',8,'SampleTime',-1,'Signal',struct('SgnName',{'FRS_P2_00_Msg_CheckSum','FRS_P2_00_Msg_AliveCounter','FRS_P2_00_Obj_MeasFlag','FRS_P2_00_Obj_YVelRel','FRS_P2_00_Obj_Type','FRS_P2_00_Obj_XPos','FRS_P2_00_Obj_YPos','FRS_P2_00_Obj_XVelRel'},'SgnStartBit',{0,8,12,13,24,26,40,53},'SgnLength',{8,4,1,11,2,14,13,11},'SgnType',{0,0,0,0,0,0,0,0},'ModeValue',{-1,-1,-1,-1,-1,-1,-1,-1},'DataType',{0,0,0,0,0,0,0,0},'ByteLayout',{2,2,2,2,2,2,2,2},'Factor',{1,1,1,0.1,1,2^-6,2^-6,0.1},'Offset',{0,0,0,-102.4,0,0,-64,-102.4},'SgnComment',{{['Check sum shall be generated out of each message content. check sum generation logic is TBC.']},{['Alive counter shall be incremented every radar sensor measurement cycle.']},{['This signal indicates whether the latest sensor measurement observed the object or extrapolated.' char(10) '0x0: object measured in this cycle' char(10) '0x1: object extrapolated in this cycle']},{['Relative lateral velocity of the object']},{['To indicate the estimated type of Object' char(10) '0x00: Unknown' char(10) '0x01: 4 wheeler' char(10) '0x02: 2 wheeler' char(10) '0x03: Pedestrian']},{['Position of target object in longitudinal direction' char(10) 'center of vehicle rear axle shaft is reference point.']},{['Position of target object in lateral direction' char(10) 'center of vehicle rear axle shaft is reference point.']},{['Relative longitudinal velocity of the object.']}},'SgnUnit',{'n/a','n/a','n/a','m/s','n/a','m','m','m/s'},'Min',{0,0,0,-102.4,0,0,-64,-102.4},'Max',{255,15,1,102.3,3,255.984375,63.984375,102.3},'SLDataType',{'SS_DOUBLE','SS_DOUBLE','SS_DOUBLE','SS_DOUBLE','SS_DOUBLE','SS_DOUBLE','SS_DOUBLE','SS_DOUBLE'}),'MsgIdNumFormat',1,'MsgComment',{{''}}),'Version',1.2,'general',struct('isFromLib',0)),'OFF',[]}},'GroupId',{{struct('Group',{{'RTICAN'}},'No',2,'Behavior',{{'NAMECHANGE'}},'BlockType',{{'SINK'}},'NameChangeFlag',0),'OFF',[]}},'SFcnRTICANMessage',{{struct('MsgType','RX','SFcnPortType','Scalar','MsgName','FRS_Obj_00_Part2of2','MsgIdFormat','STD','MsgId',32,'MsgLength',8,'NumSignals',8,'SampleTime',-1,'Signal',struct('SgnName',{'FRS_P2_00_Msg_CheckSum','FRS_P2_00_Msg_AliveCounter','FRS_P2_00_Obj_MeasFlag','FRS_P2_00_Obj_YVelRel','FRS_P2_00_Obj_Type','FRS_P2_00_Obj_XPos','FRS_P2_00_Obj_YPos','FRS_P2_00_Obj_XVelRel'},'SgnStartBit',{0,8,12,13,24,26,40,53},'SgnLength',{8,4,1,11,2,14,13,11},'SgnType',{'standard','standard','standard','standard','standard','standard','standard','standard'},'ModeValue',{-1,-1,-1,-1,-1,-1,-1,-1},'DataType',{['unsigned int'],['unsigned int'],['unsigned int'],['unsigned int'],['unsigned int'],['unsigned int'],['unsigned int'],['unsigned int']},'ByteLayout',{['motorola back.'],['motorola back.'],['motorola back.'],['motorola back.'],['motorola back.'],['motorola back.'],['motorola back.'],['motorola back.']},'Factor',{1,1,1,0.1,1,2^-6,2^-6,0.1},'Offset',{0,0,0,-102.4,0,0,-64,-102.4},'SLDataType',{'SS_DOUBLE','SS_DOUBLE','SS_DOUBLE','SS_DOUBLE','SS_DOUBLE','SS_DOUBLE','SS_DOUBLE','SS_DOUBLE'}),'StatusSelected','yes','TimeSelected','yes','DeltaTimeSelected','yes','BytePortSelected','no','MessageLengthSelected','no','TriggerPort',struct('Selected','no','TriggerType',0),'UserCoding',struct('Selected','no','InterfaceFile','UserDecodingFile','FcnName','UserDecodeFcn','InportSelected','no','InportWidth',1,'OutportSelected','no','OutportWidth',1),'EnablePortSelected','no','UseRXService','no','BoardType','DS1','BoardNo',2,'ControllerNo',1),'OFF',[]}},'TLCFileName',{{'rtican_rx_message','OFF',[]}})  RTISFcnParameters=struct('SFcnRTICANMessage','struct','TLCFileName','char')  RTIBlockParaDefault=struct('BoardTypeNo',4302,'BoardNo',1,'ChannelNo',1,'Parameters',struct('DataFileSupport',struct('DataFileSelectedMaster',0,'DataFileSelectedLocal',0,'DataFileName','','DataFileDate','','SelectedFile',['<no file selected>']),'Options',struct('StatusSelected',1,'TimeSelected',1,'DeltaTimeSelected',1,'BytePortSelected',0,'MessageLengthSelected',0,'TriggerPort',struct('Selected',0,'TriggerType','rising'),'UserCoding',struct('Selected',0,'InterfaceFile','UserDecodingFile','FcnName','UserDecodeFcn','InportSelected',0,'InportWidth',1,'OutportSelected',0,'OutportWidth',1),'EnablePortSelected',0,'SignalOnPortnameSelected',1,'UseRXService',0),'Message',struct('MsgOnBlocknameSelected',0,'MsgName',['RX Message'],'MsgIdFormat',0,'MsgId',100,'MsgLength',8,'NumSignals',1,'SampleTime',-1,'Signal',struct('SgnName',['RX signal'],'SgnStartBit',0,'SgnLength',8,'SgnType',0,'ModeValue',-1,'DataType',0,'SLDataType','SS_DOUBLE','ByteLayout',0,'Factor',1,'Offset',0,'Min',0,'Max',255,'SgnComment',{{}},'SgnUnit',''),'MsgIdNumFormat',0,'MsgComment',{{''}}),'Version',1.2,'general',struct('isFromLib',1)),'GroupId',struct('Group',{{'RTICAN'}},'No',1,'Behavior',{{'NAMECHANGE'}},'BlockType',{{'SINK'}},'NameChangeFlag',0),'SFcnRTICANMessage',struct('MsgType','RX','MsgName',['RX Message'],'MsgIdFormat','STD','MsgId',100,'MsgLength',8,'NumSignals',1,'SampleTime',-1,'Signal',struct('SgnName',['RX signal'],'SgnStartBit',0,'SgnLength',8,'SgnType','standard','ModeValue',-1,'DataType',['unsigned int'],'ByteLayout',['little endian'],'SLDataType','SS_DOUBLE','Factor',1,'Offset',0),'StatusSelected','yes','TimeSelected','yes','DeltaTimeSelected','yes','BytePortSelected','no','MessageLengthSelected','no','EnablePortSelected','no','UserCoding',struct('Selected','no','InterfaceFile','UserDecodingFile','FcnName','UserDecodeFcn','InportSelected','no','InportWidth',1,'OutportSelected','no','OutportWidth',1),'TriggerPort',struct('Selected','no','TriggerType','rising'),'UseRXService','no','BoardType','DS4302','BoardNo',1,'ControllerNo',1,'SFcnPortType','Scalar'),'TLCFileName','rtican_rx_message')
      settings: AttributesFormatString=Group Id: RTICAN2\n  SourceProductName=dSPACE RTI CAN Blockset
  Terminator3 : Terminator
  Terminator4 : Terminator
  Terminator5 : Terminator
  Out1 : Outport
  wires:
  FRS_Obj_00_Part1of2/1 -> Bus Creator1/1  "FRS_P1_00_Msg_CheckSum"
  FRS_Obj_00_Part1of2/9 -> Bus Creator1/9  "FRS_P1_00_Obj_ValidFlag"
  FRS_Obj_00_Part1of2/5 -> Bus Creator1/5  "FRS_P1_00_Obj_XAccRel"
  FRS_Obj_00_Part2of2/7 -> Bus Creator1/19  "FRS_P2_00_Obj_YPos"
  FRS_Obj_00_Part2of2/5 -> Bus Creator1/17  "FRS_P2_00_Obj_Type"
  FRS_Obj_00_Part2of2/2 -> Bus Creator1/14  "FRS_P2_00_Msg_AliveCounter"
  FRS_Obj_00_Part2of2/8 -> Bus Creator1/20  "FRS_P2_00_Obj_XVelRel"
  FRS_Obj_00_Part1of2/10 -> Bus Creator1/10  "FRS_P1_00_Obj_XPos_Stdev"
  FRS_Obj_00_Part1of2/8 -> Bus Creator1/8  "FRS_P1_00_Obj_YPos_Stdev"
  Bus Creator1/1 -> Out1/1
  FRS_Obj_00_Part2of2/3 -> Bus Creator1/15  "FRS_P2_00_Obj_MeasFlag"
  FRS_Obj_00_Part1of2/7 -> Bus Creator1/7  "FRS_P1_00_Obj_MotionPattern"
  FRS_Obj_00_Part2of2/4 -> Bus Creator1/16  "FRS_P2_00_Obj_YVelRel"
  FRS_Obj_00_Part1of2/2 -> Bus Creator1/2  "FRS_P1_00_Msg_AliveCounter"
  FRS_Obj_00_Part2of2/1 -> Bus Creator1/13  "FRS_P2_00_Msg_CheckSum"
  FRS_Obj_00_Part2of2/6 -> Bus Creator1/18  "FRS_P2_00_Obj_XPos"
  FRS_Obj_00_Part1of2/4 -> Bus Creator1/4  "FRS_P1_00_Obj_XVelRel_Stdev"
  FRS_Obj_00_Part1of2/12 -> Bus Creator1/12  "FRS_P1_00_Obj_ID"
  FRS_Obj_00_Part1of2/6 -> Bus Creator1/6  "FRS_P1_00_Obj_ObstacleProb"
  FRS_Obj_00_Part1of2/3 -> Bus Creator1/3  "FRS_P1_00_Obj_ExstProb"
  FRS_Obj_00_Part1of2/11 -> Bus Creator1/11  "FRS_P1_00_Obj_UpdateFlag"
  FRS_Obj_00_Part2of2/10 -> Terminator4/1
  FRS_Obj_00_Part2of2/9 -> Terminator3/1
  FRS_Obj_00_Part2of2/11 -> Terminator5/1
